simulink model "FSI_model_05_A_20a"  (R2024a)
settings: Solver=VariableStepAuto  StartTime=0.0  StopTime=2  MaxStep=1e-3  RelTol=1e-3
values from neighbouring files (symbols this model uses):
  cfi = 0.1    [FSI_parametry_05_A.m]
  I = 1e-4    (= 0.0001)    [FSI_parametry_05_A.m]
  L = 5e-3    (= 0.005)    [FSI_parametry_05_A.m]
  Mz = 0.02*1    (= 0.02)    [FSI_parametry_05_A.m]
  R = 20    [FSI_parametry_05_A.m]
  U = 12    [FSI_parametry_05_A.m]
settings Model: Creator=OndrejRubes  LastModifiedBy=Miloš Uhlíř
settings SolverCC: AlgebraicLoopSolver=TrustRegion
settings RTWCC: GPUComputeCapability=3.5

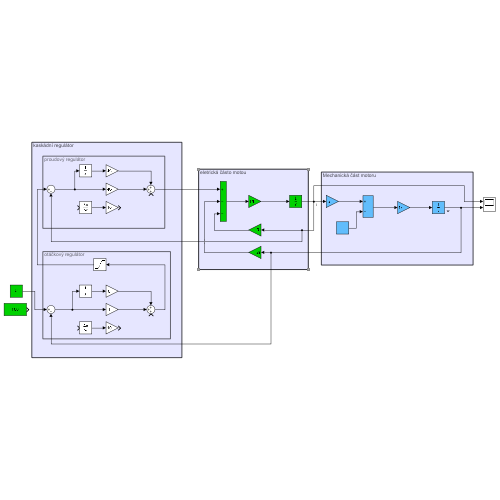
[thumbnail: Simulink's stored preview of the top-level diagram]
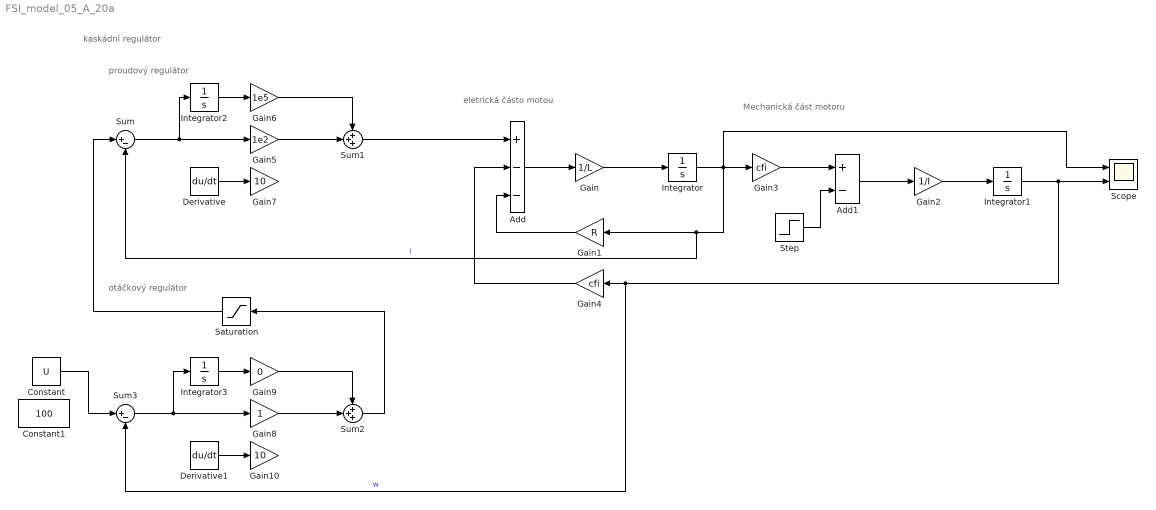
== system FSI_model_05_A_20a ==
  note: otáčkový regulátor
  note: proudový regulátor
  note: Mechanická část motoru
  note: eletrická částo motou
  note: kaskádní regulátor
  Add : Sum  Inputs=+--
  Add1 : Sum  Inputs=+-
  Constant : Constant  Value=U
  Constant1 : Constant  Value=100
  Derivative : Derivative
  Derivative1 : Derivative
  Gain : Gain  Gain=1/L
  Gain1 : Gain  Gain=R
  Gain10 : Gain  Gain=10
  Gain2 : Gain  Gain=1/I
  Gain3 : Gain  Gain=cfi
  Gain4 : Gain  Gain=cfi
  Gain5 : Gain  Gain=1e2
  Gain6 : Gain  Gain=1e5
  Gain7 : Gain  Gain=10
  Gain8 : Gain
  Gain9 : Gain  Gain=0
  Integrator{,1..3} (4 alike) : Integrator
  Saturation : Saturate
  Scope : Scope  NumInputPorts=2
  Step : Step  After=Mz  SampleTime=0
  Sum : Sum  Inputs=|+-
  Sum1 : Sum  Inputs=+++
  Sum2 : Sum  Inputs=+++
  Sum3 : Sum  Inputs=|+-
  wires:
  Gain/1 -> Integrator/1
  Add/1 -> Gain/1
  Gain1/1 -> Add/3
  Integrator/1 -> Scope/1, Gain3/1, Sum/2, Gain1/1  "i"
  Gain2/1 -> Integrator1/1
  Gain3/1 -> Add1/1
  Add1/1 -> Gain2/1
  Integrator1/1 -> Sum3/2, Gain4/1, Scope/2  "w"
  Gain4/1 -> Add/2
  Step/1 -> Add1/2
  Sum2/1 -> Saturation/1
  Derivative/1 -> Gain7/1
  Integrator2/1 -> Gain6/1
  Gain5/1 -> Sum1/2
  Gain6/1 -> Sum1/1
  Sum/1 -> Integrator2/1, Gain5/1
  Sum3/1 -> Integrator3/1, Gain8/1
  Derivative1/1 -> Gain10/1
  Gain8/1 -> Sum2/2
  Integrator3/1 -> Gain9/1
  Sum1/1 -> Add/1
  Gain9/1 -> Sum2/1
  Saturation/1 -> Sum/1
  Constant/1 -> Sum3/1
